simulink model "lab55"  (R2022b)
settings: Solver=VariableStepAuto  StartTime=0.0  StopTime=czas  MaxStep=0.1
values from neighbouring files (symbols this model uses):
  dqg = 0    [lab5.m]
  dTzew = 0    [lab5.m]
  L11 = M2    [lab5.m]
  L12 = [(Kcw*Cvp) (Kcp*Kcwp+Kcw*Kcwp+Kcw*Kcp)]    [lab5.m]
  L21 = Kcwp    (= 69.7674418605)    [lab5.m]
  L22 = [(Kcp*Cvw) (Kcwp*Kcw+Kcw*Kcp+Kcw*Kcp)]    [lab5.m]
  M = [(Cvw*Cvp) (Cvw*Kcwp+Cvw*Kcp+Cvp*Kcw+Cvp*Kcwp) (Kcw*Kcwp+Kcw*Kcp+Kcwp*Kcp)]    [lab5.m]
  t0 = 1000    [lab5.m]
  Tp0 = (Kcwp*(Kcw*Tzew0+qg0)+(Kcp*Tzew0)*(Kcw+Kcwp))/(Kcwp*Kcw+Kcp*Kcw+Kcp*Kcwp)    (= 10)    [lab5.m]
  Twew0 = (Kcw*Tzew0+Kcwp*TpN+qg0)/(Kcw+Kcwp)    (= 20)    [lab5.m]
settings Model: Creator=sebastianstanislawski  LastModifiedBy=sebastianstanislawski
settings DataIOCC: ReturnWorkspaceOutputs=off

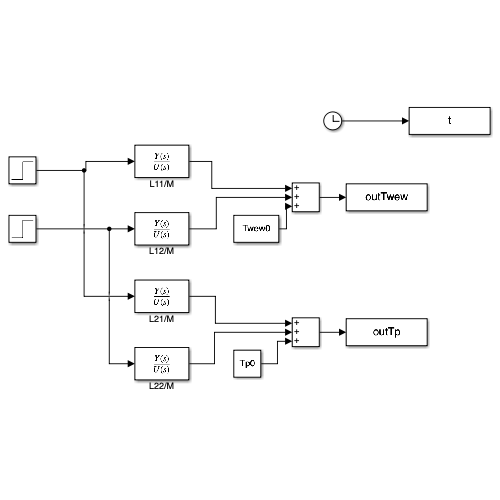
[thumbnail: Simulink's stored preview of the top-level diagram]
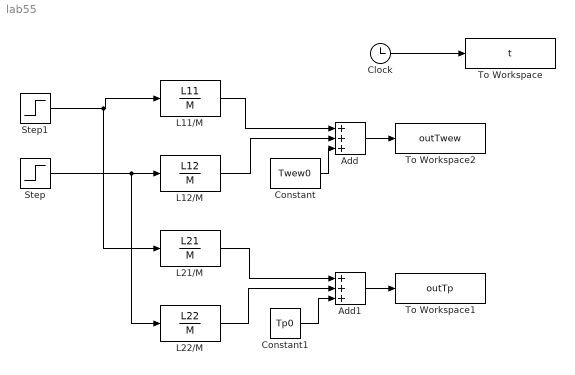
== system lab55 ==
  Add : Sum  Inputs=+++
  Add1 : Sum  Inputs=+++
  Clock : Clock
  Constant : Constant  Value=Twew0
  Constant1 : Constant  Value=Tp0
  L11/M : TransferFcn  Numerator=L11  Denominator=M
  L12/M : TransferFcn  Numerator=L12  Denominator=M
  L21/M : TransferFcn  Numerator=L21  Denominator=M
  L22/M : TransferFcn  Numerator=L22  Denominator=M
  Step : Step  Time=t0  After=dTzew  SampleTime=0
  Step1 : Step  Time=t0  After=dqg  SampleTime=0
  To Workspace : ToWorkspace  VariableName=t  SampleTime=-1
  To Workspace1 : ToWorkspace  VariableName=outTp  SampleTime=-1
  To Workspace2 : ToWorkspace  VariableName=outTwew  SampleTime=-1
  wires:
  Clock/1 -> To Workspace/1
  Step1/1 -> L21/M/1, L11/M/1
  Step/1 -> L22/M/1, L12/M/1
  L12/M/1 -> Add/2
  L11/M/1 -> Add/1
  L22/M/1 -> Add1/2
  L21/M/1 -> Add1/1
  Add1/1 -> To Workspace1/1
  Add/1 -> To Workspace2/1
  Constant/1 -> Add/3
  Constant1/1 -> Add1/3
